simulink model "GreenHydrogenMicrogrid"  (R2026a)
settings: Solver=FixedStepAuto  StopTime=24*3600*7.5  FixedStep=Ts  MaxStep=0.1  AbsTol=1e-3
PreLoadFcn:
  | GreenHydrogenMicrogridData;
values from neighbouring files (symbols this model uses):
  R_h2 = 4.12    [GreenHydrogenMicrogridData.m]
  Ts = 10    [GreenHydrogenMicrogridData.m]    (also in RL_agent.m = 1)
undefined symbols (not defined in the file or in its folder): Battery, DiscIntNeverNeededParam, Electrolyzer, Operation_Ref, Plate, Tank
libraries: fl_lib x35, nesl_utility x15, ee_lib x4, simulink x3, batteryecm_lib x1, rllib x1
(part 1 of 3)
CloseFcn:
  | try,close(h1_GreenHydrogenMicrogrid),end
  | clear h1_GreenHydrogenMicrogrid
  | 
  | 
  | clear simlog_GreenHydrogenMicrogrid
  | clear logsout_GreenHydrogenMicrogrid
  | clear T_vect h_vect nu_vect cond_vect cp_vect R_h2
  | clear t_solar_profile solar_profile temperature
  | clear Plate Electrolyzer Heat Tank H2_Tank Temp_vect_heat I_vect_heat
  | 
  | clear Battery Operation_Ref Converter Ts Ts_Control
Description:
  | Green Hydrogen Microgrid
settings Model: Creator=The MathWorks, Inc.  LastModifiedBy=shuayb
settings SolverCC: InitialStep=0.1
settings DataIOCC: SignalLoggingName=logsout_GreenHydrogenMicrogrid  OutputOption=SpecifiedOutputTimes  OutputTimes=[0:0.5:60]
settings HardwareCC: ProdHWDeviceType=32-bit Generic
settings GRTTargetCC: CombineOutputUpdateFcns=off  GRTInterface=on
settings SimscapeCC: SimscapeNormalizeSystem=off  SimscapeNominalValues="[{\"value\":\"1\",\"unit\":\"A\"},{\"value\":\"1\",\"unit\":\"bar\"},{\"value\":\"1\",\"unit\":\"cm^2\"},{\"value\":\"1\",\"unit\":\"cm^3/s\"},{\"value\":\"1\",\"unit\":\"kJ/kg\"},{\"value\":\"1\",\"unit\":\"kW\"},{\"value\":\"1\",\"unit\":\"l\"},{\"value\":\"1\",\"unit\":\"N\"},{\"value\":\"1\",\"unit\":\"N*m\"},{\"value\":\"1\",\"unit\":\"V\"}]"  SimscapeLogType=local  SimscapeLogName=simlog_GreenHydrogenMicrogrid  SimscapeLogLimitData=off

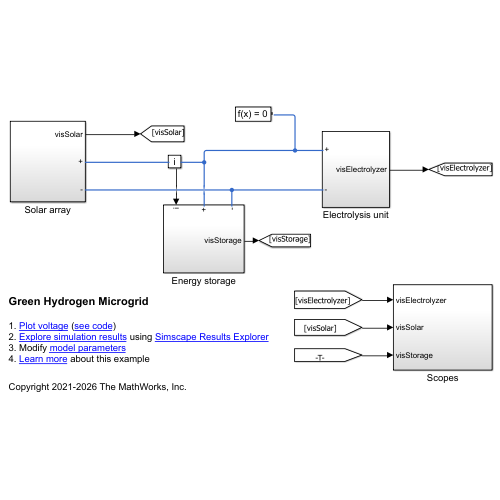
[thumbnail: Simulink's stored preview of the top-level diagram]
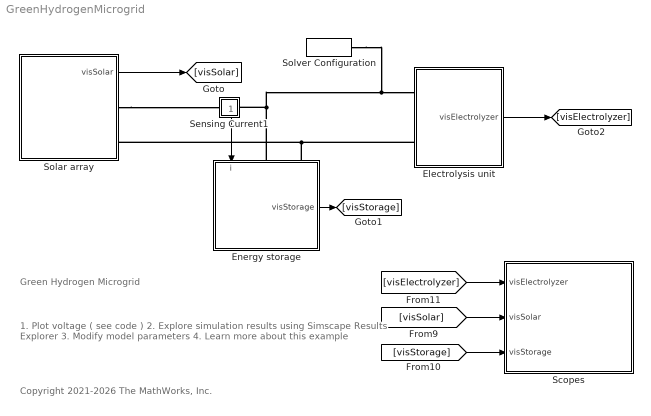
== system GreenHydrogenMicrogrid ==
  note: Green Hydrogen Microgrid
  note: 1. Plot voltage ( see code )
      | 2. Explore simulation results using Simscape Results Explorer
      | 3. Modify model parameters
      | 4. Learn more about this example
  note: Copyright 2021-2026 The MathWorks, Inc.
  Electrolysis unit : Subsystem
  Energy storage : Subsystem
      settings: PortSchema="{\"entries\":[{\"content\":{\"sides\":[{\"content\":{\"connectorIds\":[\"In1\",\"LConn1\",\"LConn2\"]},\"type\":\"ConnectorPlacement.EquallySpacedRectSide\",\"uuid\":\"9735ae67-ee5d-404d-b05d-be32c633d108\"},{\"content\":{\"connectorIds\":[],\"side\":\"RIGHT\"},\"type\":\"ConnectorPlacement.EquallySpacedRectSide\",\"uuid\":\"d60100ac-ad33-48fb-ae9c-ece9d5c3c2d8\"},{\"content\":{\"connectorIds\":[],\"side\":\"TOP\"},\"type\":\"ConnectorPlacement.EquallySpacedRectSide\",\"uuid\":\"bd9309c3-1d63-4562-a913-d4153a459f8d\"},{\"content\":{\"connectorIds\":[\"Out1\"],\"side\":\"BOTTOM\"},\"type\":\"ConnectorPlacement.EquallySpacedRectSide\",\"uuid\":\"c79ca6fd-7387-49b3-8319-60af1e13318c\"}]},\"type\":\"ConnectorPlacement.EquallySpacedConnector\",\"uuid\":\"651f9e49-8fa0-4748-8143-2e78a4ef26c5\"}],\"packageUris\":[\"http://schema.mathworks.com/mf0/Connector/R2020b\"],\"version\":\"1.0\"}"
  Scopes : Subsystem
  Sensing Current1 : Subsystem
      settings: PortSchema="{\"entries\":[{\"content\":{\"sides\":[{\"content\":{\"connectorIds\":[\"LConn1\"]},\"type\":\"ConnectorPlacement.EquallySpacedRectSide\",\"uuid\":\"e3c1304f-b602-4c8c-83ae-2fd3882be16e\"},{\"content\":{\"connectorIds\":[\"RConn1\"],\"side\":\"RIGHT\"},\"type\":\"ConnectorPlacement.EquallySpacedRectSide\",\"uuid\":\"8d7546a0-f580-4754-b3ac-0546585847f9\"},{\"content\":{\"connectorIds\":[],\"side\":\"TOP\"},\"type\":\"ConnectorPlacement.EquallySpacedRectSide\",\"uuid\":\"be7a685a-381b-4438-acf4-f99982fa8e59\"},{\"content\":{\"connectorIds\":[\"Out1\"],\"side\":\"BOTTOM\"},\"type\":\"ConnectorPlacement.EquallySpacedRectSide\",\"uuid\":\"49077b64-a22b-4a01-86bf-86bb36c1b22f\"}]},\"type\":\"ConnectorPlacement.EquallySpacedConnector\",\"uuid\":\"e35d636b-ea96-4c19-a517-3c12fcbe0b84\"}],\"packageUris\":[\"http://schema.mathworks.com/mf0/Connector/R2020b\"],\"version\":\"1.0\"}"
      mask Display: disp('i')
  Solar array : Subsystem
  Solver Configuration : nesl_utility/Solver Configuration  PhysicalDomain=network_engine_domain  SubClassName=solver  LeftPortType=input  RightPortType=generic  Tones=[]  Harmonics=[]  SimulateNoise=off  Profile=off  UseLocalSampling=off  EnableSwitchedLinearOptims=on  FrequencyDomain=off  UseCCode=off  RelTol=0.001  AbsTol=1e-06  MinStep=1e-09  ToWorkspace=off  RevertToSquareIcSolve=off  NumHomotopyIterations=100  PhasorMode=off  PhasorModeNumHarmonics=1  ConsistencySolver=NEWTON_FTOL  CanonicalOrdering=UNORDERED  OptimizeIntermediates=UNOPTIMIZED  IndexReductionMethod=DerivativeReplacement  DoDC=off  ResidualTolerance=1e-9  ConsistencyTolSource=GLOBAL  ConsistencyAbsTol=0.001  ConsistencyRelTol=0.001  ConsistencyTolFactor=0.001  UseLocalSolver=on  LocalSolverChoice=NE_BACKWARD_EULER_ADVANCER  ResolveIndetEquations=on  FunctionEvalNumThread=1  LocalSolverSampleTime=Ts  DoFixedCost=on  MaxNonlinIter=3  MaxModeIter=2  ComputeImpulses=off  ImpulseIterations=2  LinearAlgebra=auto  LinearAlgebraNumThread=0  EquationFormulation=NE_TIME_EF  DelaysMemoryBudget=1024  AutomaticFiltering=on  FilteringTimeConstant=0.001  PartitionStorageMethod=AS_NEEDED  PartitionMemoryBudget=1024  PartitionMethod=FAST  MultibodyUseLocalSolver=off  MultibodyLocalSolverChoice=ODE1  MultibodyLocalSolverSampleTime=0.001
  wires:
  Sensing Current1/1(iout) -> Energy storage/1(i)
  Solar array/1(visSolar) -> [visSolar]
  Energy storage/1(visStorage) -> [visStorage]
  Electrolysis unit/1(visElectrolyzer) -> [visElectrolyzer]
  [visSolar] -> Scopes/2(visSolar)
  [visElectrolyzer] -> Scopes/1(visElectrolyzer)
  [visStorage] -> Scopes/3(visStorage)
  connections:
  Energy storage/LConn2 -- Electrolysis unit/LConn2 -- Solar array/RConn2
  Energy storage/LConn1 -- Sensing Current1/RConn1 -- Solver Configuration/RConn1 -- Electrolysis unit/LConn1
  Solar array/RConn1 -- Sensing Current1/LConn1
